simulink model "BatteryModel"  (R2026b)
settings: Solver=ode45  StopTime=1
undefined symbols (not defined in the file): Battery
settings Model: DataDictionary=VehicleData.sldd  Creator=Xu Dingyi  LastModifiedBy=29358

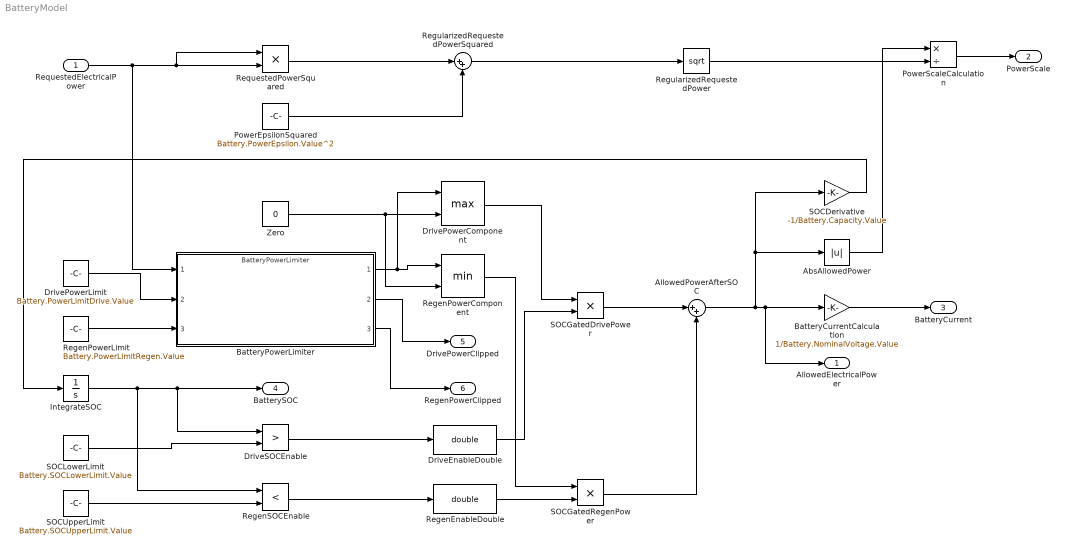
== system BatteryModel ==
  RequestedElectricalPower : Inport  OutDataTypeStr=double  PortDimensions=1
  AbsAllowedPower : Abs
  AllowedPowerAfterSOC : Sum  Inputs=|++
  BatteryCurrentCalculation : Gain  Gain=1/Battery.NominalVoltage.Value
  BatteryPowerLimiter : ModelReference  ModelNameDialog=BatteryPowerLimiter  SimulationMode=Normal  ModelReferenceVersion=1.1
  DriveEnableDouble : DataTypeConversion  OutDataTypeStr=double
  DrivePowerComponent : MinMax  Function=max  Inputs=2
  DrivePowerLimit : Constant  Value=Battery.PowerLimitDrive.Value  OutDataTypeStr=double
  DriveSOCEnable : RelationalOperator  Operator=>
  IntegrateSOC : Integrator  InitialCondition=Battery.InitialSOC.Value  LimitOutput=on  UpperSaturationLimit=1  LowerSaturationLimit=0
  PowerEpsilonSquared : Constant  Value=Battery.PowerEpsilon.Value^2  OutDataTypeStr=double
  PowerScaleCalculation : Product  Inputs=*/
  RegenEnableDouble : DataTypeConversion  OutDataTypeStr=double
  RegenPowerComponent : MinMax  Inputs=2
  RegenPowerLimit : Constant  Value=Battery.PowerLimitRegen.Value  OutDataTypeStr=double
  RegenSOCEnable : RelationalOperator  Operator=<
  RegularizedRequestedPower : Sqrt
  RegularizedRequestedPowerSquared : Sum  Inputs=|++
  RequestedPowerSquared : Product  Inputs=**
  SOCDerivative : Gain  Gain=-1/Battery.Capacity.Value
  SOCGatedDrivePower : Product  Inputs=**
  SOCGatedRegenPower : Product  Inputs=**
  SOCLowerLimit : Constant  Value=Battery.SOCLowerLimit.Value  OutDataTypeStr=double
  SOCUpperLimit : Constant  Value=Battery.SOCUpperLimit.Value  OutDataTypeStr=double
  Zero : Constant  Value=0  OutDataTypeStr=double
  AllowedElectricalPower : Outport
  PowerScale : Outport  Port=2
  BatteryCurrent : Outport  Port=3
  BatterySOC : Outport  Port=4
  DrivePowerClipped : Outport  Port=5
  RegenPowerClipped : Outport  Port=6
  wires:
  BatteryPowerLimiter/3 -> RegenPowerClipped/1
  BatteryPowerLimiter/2 -> DrivePowerClipped/1
  BatteryCurrentCalculation/1 -> BatteryCurrent/1
  RegularizedRequestedPower/1 -> PowerScaleCalculation/2
  AbsAllowedPower/1 -> PowerScaleCalculation/1
  RegularizedRequestedPowerSquared/1 -> RegularizedRequestedPower/1
  PowerEpsilonSquared/1 -> RegularizedRequestedPowerSquared/2
  RequestedPowerSquared/1 -> RegularizedRequestedPowerSquared/1
  SOCDerivative/1 -> IntegrateSOC/1
  AllowedPowerAfterSOC/1 -> BatteryCurrentCalculation/1, AllowedElectricalPower/1, SOCDerivative/1, AbsAllowedPower/1
  SOCGatedRegenPower/1 -> AllowedPowerAfterSOC/2
  SOCGatedDrivePower/1 -> AllowedPowerAfterSOC/1
  RegenEnableDouble/1 -> SOCGatedRegenPower/2
  RegenPowerComponent/1 -> SOCGatedRegenPower/1
  DriveEnableDouble/1 -> SOCGatedDrivePower/2
  DrivePowerComponent/1 -> SOCGatedDrivePower/1
  RegenSOCEnable/1 -> RegenEnableDouble/1
  DriveSOCEnable/1 -> DriveEnableDouble/1
  SOCUpperLimit/1 -> RegenSOCEnable/2
  SOCLowerLimit/1 -> DriveSOCEnable/2
  IntegrateSOC/1 -> DriveSOCEnable/1, BatterySOC/1, RegenSOCEnable/1
  Zero/1 -> DrivePowerComponent/2, RegenPowerComponent/2
  BatteryPowerLimiter/1 -> DrivePowerComponent/1, RegenPowerComponent/1
  RegenPowerLimit/1 -> BatteryPowerLimiter/3
  DrivePowerLimit/1 -> BatteryPowerLimiter/2
  RequestedElectricalPower/1 -> RequestedPowerSquared/1, RequestedPowerSquared/2, BatteryPowerLimiter/1
  PowerScaleCalculation/1 -> PowerScale/1
